simulink model "main_vehicle_v2"  (R2024b)
settings: Solver=FixedStepAuto  StartTime=0.0  StopTime=60  FixedStep=Ts  RelTol=1e-3
values from neighbouring files (symbols this model uses):
  Frr = Crr*m*g    (= 53.955)    [main_data_vehicle.m]
  v0 = 10    [main_data_vehicle.m]
settings Model: Creator=marti  LastModifiedBy=marti

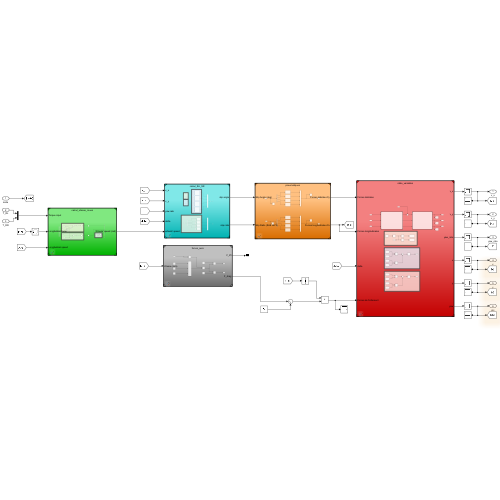
[thumbnail: Simulink's stored preview of the top-level diagram]
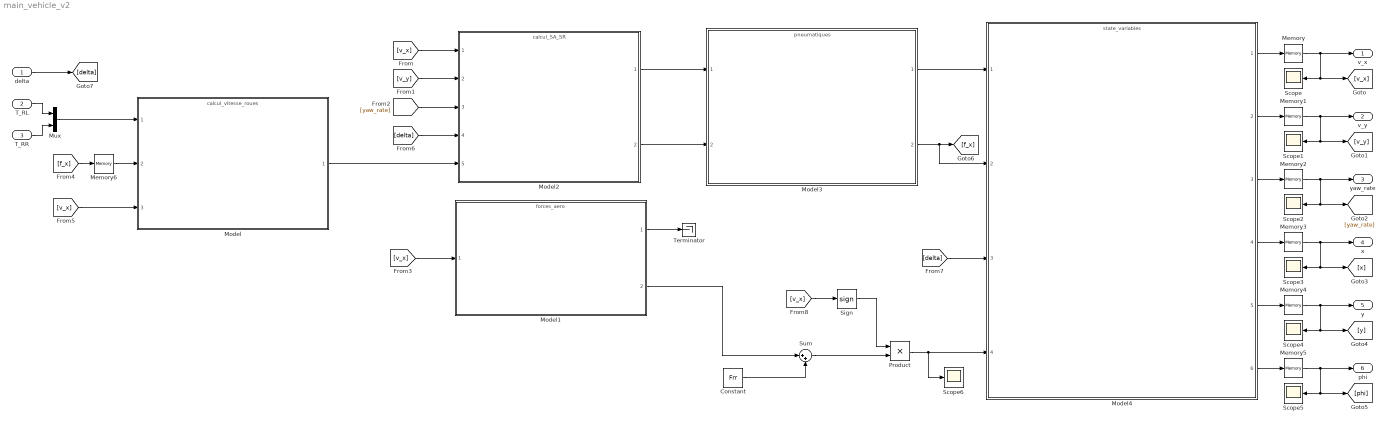
== system main_vehicle_v2 ==
  delta : Inport
  T_RL : Inport  Port=2
  T_RR : Inport  Port=3
  Constant : Constant  Value=Frr
  Memory : Memory  InitialCondition=v0
  Memory{1..5} (5 alike) : Memory
  Memory6 : Memory  InitialCondition=[0 0 0 0]
  Model : ModelReference  ModelNameDialog=calcul_vitesse_roues.slx  SimulationMode=Normal  ModelReferenceVersion=1.23
  Model1 : ModelReference  ModelNameDialog=forces_aero.slx  SimulationMode=Normal  ModelReferenceVersion=1.4
  Model2 : ModelReference  ModelNameDialog=calcul_SA_SR.slx  SimulationMode=Normal  ModelReferenceVersion=1.27
  Model3 : ModelReference  ModelNameDialog=pneumatiques.slx  SimulationMode=Normal  ModelReferenceVersion=1.26
  Model4 : ModelReference  ModelNameDialog=state_variables.slx  SimulationMode=Normal  ModelReferenceVersion=1.3
  Mux : Mux  Inputs=2
  Product : Product
  Scope{,1..6} (7 alike) : Scope
  Sign : Signum
  Sum : Sum  Inputs=|++
  Terminator : Terminator
  v_x : Outport
  v_y : Outport  Port=2
  yaw_rate : Outport  Port=3
  x : Outport  Port=4
  y : Outport  Port=5
  phi : Outport  Port=6
  wires:
  Model2/1 -> Model3/1
  Model2/2 -> Model3/2
  Model3/1 -> Model4/1
  Model3/2 -> Model4/2, [f_x]
  Model4/1 -> Memory/1
  Model4/2 -> Memory1/1
  Model4/3 -> Memory2/1
  Model4/4 -> Memory3/1
  Model4/5 -> Memory4/1
  Model4/6 -> Memory5/1
  [v_x] -> Model2/1
  [v_y] -> Model2/2
  [yaw_rate] -> Model2/3
  Model/1 -> Model2/5
  [v_x] -> Model1/1
  [f_x] -> Memory6/1
  [v_x] -> Model/3
  [delta] -> Model2/4
  [delta] -> Model4/3
  Model1/1 -> Terminator/1
  Constant/1 -> Sum/2
  Model1/2 -> Sum/1
  [v_x] -> Sign/1
  Sum/1 -> Product/2
  Sign/1 -> Product/1
  Memory/1 -> v_x/1, Scope/1, [v_x]
  Memory1/1 -> v_y/1, Scope1/1, [v_y]
  Memory2/1 -> yaw_rate/1, [yaw_rate], Scope2/1
  Memory3/1 -> x/1, Scope3/1, [x]
  Memory4/1 -> y/1, [y], Scope4/1
  Memory5/1 -> phi/1, Scope5/1, [phi]
  Product/1 -> Scope6/1, Model4/4
  delta/1 -> [delta]
  T_RL/1 -> Mux/1
  T_RR/1 -> Mux/2
  Mux/1 -> Model/1
  Memory6/1 -> Model/2
